simulink model "CSA_VSI"  (R2024b)
settings: Solver=FixedStepAuto  StartTime=0.0  StopTime=Inf  RelTol=1e-3  EnableMultiTasking=on
InitFcn:
  | iq_openloop = 2;
  | vq_openloop = 0.1;
  | SFOL = 1;
  | FOL = 10;
  | Alignment = 0;
  | ModulationStrategy = 1;
  | DPWM1 = 1;
  | DPWM2 = 1;
  | da = 1;
  | db = 0;
  | dc = 0;
  | uab = 1;
  | ubc = 1;
  | iab = 1;
  | ibc = 1;
  | swi = 1;
  | wref_input = 100;
values from neighbouring files (symbols this model uses):
  bus = 400    [CSA_VSI_param.m]
  d0 = 0    [CSA_VSI_param.m]
  k = 2e-4    (= 0.0002)    [CSA_VSI_param.m]
  ki = 94.6    [CSA_VSI_param.m]
  PWM_timer_123 = int32(F_dsp/(2*Fs_1))    [CSA_VSI_param.m]
  slope = 100    [CSA_VSI_param.m]
  Ts_1 = 1/Fs_1    (= 1e-05)    [CSA_VSI_param.m]
  Vref = 100    [CSA_VSI_param.m]
  VrefFreq = 60    [CSA_VSI_param.m]
undefined symbols (not defined in the file or in its folder): DiscIntNeverNeededParam, Down, GPTRIP1SEL, GPTRIP2SEL, TZ1, TZ2, Up
libraries: c2802xlib x13, simulink x11, c2837xDlib x6, simulink_extras x2, c2000lib x1, idelinklib_common x1
(part 2 of 2)

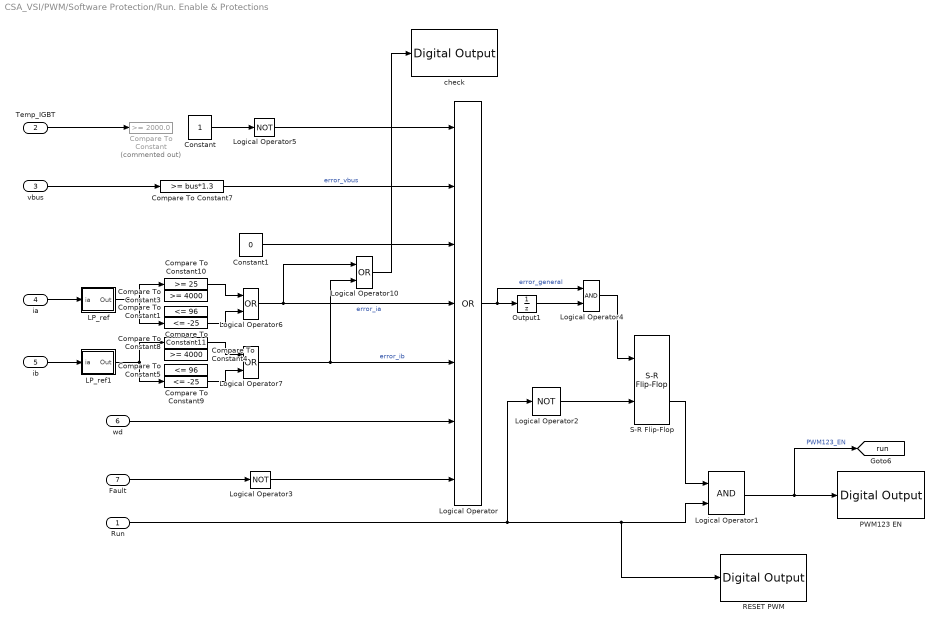
== system CSA_VSI/PWM/Software Protection/Run. Enable & Protections ==
  Run : Inport
  Temp_IGBT : Inport  Port=2
  vbus : Inport  Port=3
  ia : Inport  Port=4
  ib : Inport  Port=5
  wd : Inport  Port=6
  Fault : Inport  Port=7
  Compare To Constant : simulink/Logic and Bit Operations/Compare To Constant  Commented=on  relop=>=  const=2000.0  OutDataTypeStr=boolean
  Compare To Constant1 : simulink/Logic and Bit Operations/Compare To Constant  relop=<=  const=96  OutDataTypeStr=boolean
  Compare To Constant10 : simulink/Logic and Bit Operations/Compare To Constant  relop=>=  const=25  OutDataTypeStr=boolean
  Compare To Constant11 : simulink/Logic and Bit Operations/Compare To Constant  relop=<=  const=-25  OutDataTypeStr=boolean
  Compare To Constant3 : simulink/Logic and Bit Operations/Compare To Constant  relop=>=  const=4000  OutDataTypeStr=boolean
  Compare To Constant4 : simulink/Logic and Bit Operations/Compare To Constant  relop=>=  const=4000  OutDataTypeStr=boolean
  Compare To Constant5 : simulink/Logic and Bit Operations/Compare To Constant  relop=<=  const=96  OutDataTypeStr=boolean
  Compare To Constant7 : simulink/Logic and Bit Operations/Compare To Constant  relop=>=  const=bus*1.3  OutDataTypeStr=boolean
  Compare To Constant8 : simulink/Logic and Bit Operations/Compare To Constant  relop=>=  const=25  OutDataTypeStr=boolean
  Compare To Constant9 : simulink/Logic and Bit Operations/Compare To Constant  relop=<=  const=-25  OutDataTypeStr=boolean
  Constant : Constant  OutDataTypeStr=boolean
  Constant1 : Constant  Value=0  OutDataTypeStr=boolean
  LP_ref : Subsystem
  LP_ref1 : Subsystem
  Logical Operator : Logic  Operator=OR  Inputs=7  AllPortsSameDT=off  OutDataTypeStr=boolean
  Logical Operator1 : Logic  AllPortsSameDT=off  OutDataTypeStr=boolean
  Logical Operator10 : Logic  Operator=OR  AllPortsSameDT=off  OutDataTypeStr=boolean
  Logical Operator2 : Logic  Operator=NOT  Inputs=1  AllPortsSameDT=off  OutDataTypeStr=boolean
  Logical Operator3 : Logic  Operator=NOT  Inputs=1  AllPortsSameDT=off  OutDataTypeStr=boolean
  Logical Operator4 : Logic  AllPortsSameDT=off  OutDataTypeStr=boolean
  Logical Operator5 : Logic  Operator=NOT  Inputs=1  AllPortsSameDT=off  OutDataTypeStr=boolean
  Logical Operator6 : Logic  Operator=OR  AllPortsSameDT=off  OutDataTypeStr=boolean
  Logical Operator7 : Logic  Operator=OR  AllPortsSameDT=off  OutDataTypeStr=boolean
  Output1 : UnitDelay  SampleTime=-1  HasFrameUpgradeWarning=on
  PWM123 EN : c2837xDlib/Digital Output  GPIO_Number=GPIO16~GPIO23  GPIO_Bit0=off  GPIO_BIT0_Toggle=off  GPIO_Bit1=off  GPIO_BIT1_Toggle=off  GPIO_Bit2=on  GPIO_BIT2_Toggle=off  GPIO_Bit3=off  GPIO_BIT3_Toggle=off  GPIO_Bit4=off  GPIO_BIT4_Toggle=off  GPIO_Bit5=off  GPIO_BIT5_Toggle=off  GPIO_Bit6=off  GPIO_BIT6_Toggle=off  GPIO_Bit7=off  GPIO_BIT7_Toggle=off
  RESET PWM : c2837xDlib/Digital Output  GPIO_Number=GPIO88~GPIO95  GPIO_Bit0=off  GPIO_BIT0_Toggle=off  GPIO_Bit1=off  GPIO_BIT1_Toggle=off  GPIO_Bit2=off  GPIO_BIT2_Toggle=off  GPIO_Bit3=off  GPIO_BIT3_Toggle=off  GPIO_Bit4=off  GPIO_BIT4_Toggle=off  GPIO_Bit5=off  GPIO_BIT5_Toggle=off  GPIO_Bit6=on  GPIO_BIT6_Toggle=off  GPIO_Bit7=off  GPIO_BIT7_Toggle=off
  S-R Flip-Flop : simulink_extras/Flip Flops/S-R Flip-Flop  initial_condition=1
  check : c2837xDlib/Digital Output  GPIO_Number=GPIO104~GPIO111  GPIO_Bit0=on  GPIO_BIT0_Toggle=off  GPIO_Bit1=off  GPIO_BIT1_Toggle=off  GPIO_Bit2=off  GPIO_BIT2_Toggle=off  GPIO_Bit3=off  GPIO_BIT3_Toggle=off  GPIO_Bit4=off  GPIO_BIT4_Toggle=off  GPIO_Bit5=off  GPIO_BIT5_Toggle=off  GPIO_Bit6=off  GPIO_BIT6_Toggle=off  GPIO_Bit7=off  GPIO_BIT7_Toggle=off
  tag scope: run=global
  wires:
  Logical Operator2/1 -> S-R Flip-Flop/2
  S-R Flip-Flop/2 -> Logical Operator1/1
  Fault/1 -> Logical Operator3/1
  Logical Operator1/1 -> PWM123 EN/1, [run]  "PWM123_EN"
  vbus/1 -> Compare To Constant7/1
  Logical Operator5/1 -> Logical Operator/1
  Compare To Constant7/1 -> Logical Operator/2  "error_vbus"
  Constant1/1 -> Logical Operator/3
  Logical Operator6/1 -> Logical Operator10/1, Logical Operator/4  "error_ia"
  Logical Operator7/1 -> Logical Operator10/2, Logical Operator/5  "error_ib"
  wd/1 -> Logical Operator/6
  Logical Operator3/1 -> Logical Operator/7
  Temp_IGBT/1 -> Compare To Constant/1
  Output1/1 -> Logical Operator4/2
  Logical Operator/1 -> Logical Operator4/1, Output1/1  "error_general"
  Logical Operator4/1 -> S-R Flip-Flop/1
  Constant/1 -> Logical Operator5/1
  LP_ref/1(Out) -> Compare To Constant11/1, Compare To Constant10/1
  LP_ref1/1(Out) -> Compare To Constant9/1, Compare To Constant8/1
  Compare To Constant10/1 -> Logical Operator6/1
  Compare To Constant11/1 -> Logical Operator6/2
  Compare To Constant8/1 -> Logical Operator7/1
  Compare To Constant9/1 -> Logical Operator7/2
  ia/1 -> LP_ref/1(ia)
  ib/1 -> LP_ref1/1(ia)
  Run/1 -> RESET PWM/1, Logical Operator1/2, Logical Operator2/1
  Logical Operator10/1 -> check/1

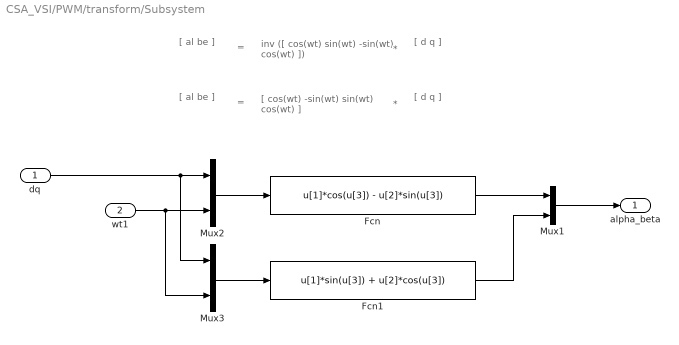
== system CSA_VSI/PWM/transform/Subsystem ==
  note: inv ([  cos(wt)   sin(wt)
      |    -sin(wt)    cos(wt)   ])
  note: *
  note: =
  note: [  al
      |     be  ]
  note: =
  note: [ d
      |    q ]
  note: [  al
      |     be  ]
  note: [ d
      |    q ]
  note: *
  note: [  cos(wt)   -sin(wt)
      |    sin(wt)    cos(wt)   ]
  dq : Inport  PortDimensions=2
  wt1 : Inport  Port=2  PortDimensions=1
  Fcn : Fcn  Expr=u[1]*cos(u[3]) - u[2]*sin(u[3])
  Fcn1 : Fcn  Expr=u[1]*sin(u[3]) + u[2]*cos(u[3])
  Mux1 : Mux  Inputs=2
  Mux2 : Mux  Inputs=[2 1]
  Mux3 : Mux  Inputs=[2 1]
  alpha_beta : Outport  InitialOutput=[0,0]  VectorParamsAs1DForOutWhenUnconnected=off
  wires:
  wt1/1 -> Mux3/2, Mux2/2
  Mux1/1 -> alpha_beta/1
  Mux2/1 -> Fcn/1
  Mux3/1 -> Fcn1/1
  Fcn1/1 -> Mux1/2
  Fcn/1 -> Mux1/1
  dq/1 -> Mux3/1, Mux2/1

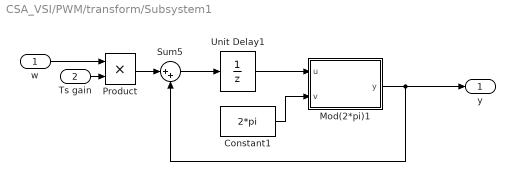
== system CSA_VSI/PWM/transform/Subsystem1 ==
  w : Inport
  Ts gain : Inport  Port=2  OutDataTypeStr=single
  Constant1 : Constant  Value=2*pi  VectorParams1D=off  OutDataTypeStr=single
  Mod(2*pi)1 : MATLAB Function  TreatAsAtomicUnit=on
  Product : Product  OutDataTypeStr=single
  Sum5 : Sum  Inputs=|++
  Unit Delay1 : UnitDelay  SampleTime=-1
  y : Outport  OutDataTypeStr=single
  wires:
  Mod(2*pi)1/1(y) -> y/1, Sum5/2
  Unit Delay1/1 -> Mod(2*pi)1/1(u)
  Sum5/1 -> Unit Delay1/1
  Constant1/1 -> Mod(2*pi)1/2(v)
  Product/1 -> Sum5/1
  w/1 -> Product/1
  Ts gain/1 -> Product/2

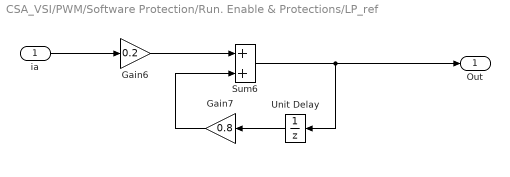
== system CSA_VSI/PWM/Software Protection/Run. Enable & Protections/LP_ref ==
  ia : Inport
  Gain6 : Gain  Gain=0.2  ParamDataTypeStr=single  OutDataTypeStr=single  RndMeth=Zero
  Gain7 : Gain  Gain=0.8  ParamDataTypeStr=single  OutDataTypeStr=single  RndMeth=Zero
  Sum6 : Sum  OutDataTypeStr=int32  AccumDataTypeStr=single  RndMeth=Zero
  Unit Delay : UnitDelay  SampleTime=-1  HasFrameUpgradeWarning=on
  Out : Outport  VectorParamsAs1DForOutWhenUnconnected=off
  wires:
  ia/1 -> Gain6/1
  Sum6/1 -> Out/1, Unit Delay/1
  Gain6/1 -> Sum6/1
  Unit Delay/1 -> Gain7/1
  Gain7/1 -> Sum6/2

== system CSA_VSI/PWM/Software Protection/Run. Enable & Protections/LP_ref1 ==
  ia : Inport
  Gain6 : Gain  Gain=0.2  ParamDataTypeStr=single  OutDataTypeStr=single  RndMeth=Zero
  Gain7 : Gain  Gain=0.8  ParamDataTypeStr=single  OutDataTypeStr=single  RndMeth=Zero
  Sum6 : Sum  OutDataTypeStr=int32  AccumDataTypeStr=single  RndMeth=Zero
  Unit Delay : UnitDelay  SampleTime=-1  HasFrameUpgradeWarning=on
  Out : Outport  VectorParamsAs1DForOutWhenUnconnected=off
  wires:
  Gain7/1 -> Sum6/2
  Unit Delay/1 -> Gain7/1
  Gain6/1 -> Sum6/1
  Sum6/1 -> Unit Delay/1, Out/1
  ia/1 -> Gain6/1

== matlab function CSA_VSI/PWM/SBI/SECTOR BASED IMPLEMENTATION ==
  data: uph input; u_SBI output; SECTOR output; PWM_timer_123 input
function [u_SBI,SECTOR]  = SBI(uph,PWM_timer_123)
u_SBI=[PWM_timer_123;PWM_timer_123;PWM_timer_123];
SECTOR=0;


if uph<=30 && uph>-30 % SECTOR 1
u_SBI=[PWM_timer_123;0;0];
SECTOR=1;
elseif uph>30 && uph<=90 % SECTOR 2
u_SBI=[PWM_timer_123;PWM_timer_123;0];
SECTOR=2;
elseif uph>90 && uph<=150  % SECTOR 3        
u_SBI=[0;PWM_timer_123;0];
SECTOR=3;
elseif (uph>150 && uph<=180) || (uph>=-180 && uph<=-150) % SECTOR 4
u_SBI=[0;PWM_timer_123;PWM_timer_123];
SECTOR=4;
elseif uph>-150 && uph<=-90 % SECTOR 5
u_SBI=[0;0;PWM_timer_123];
SECTOR=5;
elseif uph>-90 && uph<=-30 % SECTOR 6
u_SBI=[PWM_timer_123;0;PWM_timer_123];
SECTOR=6;
else
    u_SBI=[PWM_timer_123;PWM_timer_123;PWM_timer_123];
end
end

== matlab function CSA_VSI/PWM/transform/Subsystem1/Mod(2*pi)1 ==
  data: u input; y output; v input
function y = Mod_2_pi(u,v)
%#eml
if (u < v)
    y = u;
else
    y=u-v;
end

== matlab function CSA_VSI/PWM/w_ref dv//dt Limiter ==
  data: wref_ele input; slope input; wref1_ele output; en input
function wref1_ele = fcn(wref_ele,slope,en)
%#eml

persistent w;
if isempty(w) w=single(0); end

if en==1
    if w>wref_ele
        wref1_ele=single(w-slope);  
    elseif w<wref_ele
        wref1_ele=single(w+slope);  
    else 
        wref1_ele=single(w);
    end
else
    wref1_ele=single(0);
end

w=single(wref1_ele);

== matlab function CSA_VSI/PWM/ZCSMC/ZERO-VECTOR COMPLEX SLIDING MODULATION ==
  data: uph input; TimerPeriod input; ua output single; ub output; uc output; SECTOR output; d0 input
function [ua,ub,uc,SECTOR]  = zCSM(uph,TimerPeriod, d0)
uon=single(TimerPeriod-0);
uoff=single(0);
ua=uoff; ub=uoff; uc=uoff;
% d0=0;
SECTOR=0;


% SECTOR 1
if uph<=60 && uph>0
d=(uph-0)*0.016666666666667;
%d0=sqrt(d*d-d+1)-0.866;
da=(1-d0)*d;
ua=(1-d0)*TimerPeriod; ub=da*TimerPeriod; uc=uoff;
%ua=da*TimerPeriod; ub=(1-d0)*TimerPeriod; uc=uoff;
SECTOR=1;
end

% SECTOR 2
if uph>60 && uph<=120
d=(uph-60)*0.016666666666667;
%d0=sqrt(d*d-d+1)-0.866;
da=(1-d0)*d;
ua=(1-da)*TimerPeriod; ub=uon; uc=d0*TimerPeriod;
%ua=d0*TimerPeriod; ub=uon; uc=(1-da)*TimerPeriod;
SECTOR=2;
end
                    
% SECTOR 3
if uph>120 && uph<=180 %(uph<=180 || uph<=-180)
d=(uph-120)*0.016666666666667;
%d0=sqrt(d*d-d+1)-0.866;
da=(1-d0)*d;
ua=uoff; ub=(1-d0)*TimerPeriod; uc=da*TimerPeriod;  
%ua=uoff; ub=da*TimerPeriod; uc=(1-d0)*TimerPeriod;
SECTOR=3;
end

% SECTOR 4
if uph>=-180 && uph<=-120
d=(uph--180)*0.016666666666667;
%d0=sqrt(d*d-d+1)-0.866;
da=(1-d0)*d;
ua=d0*TimerPeriod; ub=(1-da)*TimerPeriod; uc=uon;
%ua=(1-da)*TimerPeriod; ub=d0*TimerPeriod; uc=uon;
SECTOR=4;
end

% SECTOR 5
if uph>-120 && uph<=-60
d=(uph--120)*0.016666666666667;
%d0=sqrt(d*d-d+1)-0.866;
da=(1-d0)*d;
ua=da*TimerPeriod; ub=uoff; uc=(1-d0)*TimerPeriod;
%ua=(1-d0)*TimerPeriod; ub=uoff; uc=da*TimerPeriod;
SECTOR=5;
end

% SECTOR 6
if uph>-60 && uph<=0
d=(uph--60)*0.016666666666667;
%d0=sqrt(d*d-d+1)-0.866;
da=(1-d0)*d;
ua=uon; ub=d0*TimerPeriod; uc=(1-da)*TimerPeriod;
%ua=uon; ub=(1-da)*TimerPeriod; uc=d0*TimerPeriod;
SECTOR=6;
end

end
